simulink model "KDO"  (R2017b)
settings: Solver=FixedStepAuto  StartTime=0.0  StopTime=100  FixedStep=0.001  RelTol=1e-3
undefined symbols (not defined in the file or in its folder): B, k1, k2, k3, k4, k5, k6, MI
libraries: powerlib_extras x15, commchan3 x15, simulink x3, checkpacklib x1
(part 1 of 3)
settings Model: Creator=Jose_Canche  LastModifiedBy=nuradeen
settings DataIOCC: LimitDataPoints=on  SaveFormat=Array
settings OptimizationCC: ExpressionDepthLimit=2147483647  InitFltsAndDblsToZero=on  LifeSpan=inf
settings DebuggingCC: SaveWithParameterizedLinksMsg=none  UnderspecifiedInitializationDetection=Classic  MergeDetectMultiDrivingBlocksExec=none  SolverPrmCheckMsg=warning  FcnCallInpInsideContextMsg=warning  StateNameClashWarn=warning  SFUnexpectedBacktrackingDiag=warning  SFNoUnconditionalDefaultTransitionDiag=warning  SFExecutionAtInitializationDiag=none
settings HardwareCC: ProdBitPerPointer=32  ProdBitPerSizeT=32  ProdBitPerPtrDiffT=32  ProdLargestAtomicFloat=None  ProdIntDivRoundTo=Undefined  ProdEndianess=Unspecified  ProdWordSize=32  ProdHWDeviceType=32-bit Generic
settings ModelReferenceCC: PropagateSignalLabelsOutOfModel=off
settings SFSimCC: SimParseCustomCode=off
settings CodeAppCC: StateflowObjectComments=on
settings GRTTargetCC: TargetFcnLib=ansi_tfl_tmw.mat  TargetLangStandard=C89/C90 (ANSI)  GeneratePreprocessorConditionals=Disable all  CombineOutputUpdateFcns=off  GRTInterface=on
settings ConfigComp: CovMetricSettings=dw  CovHtmlReporting=on  CovSaveCumulativeToWorkspaceVar=on  CovSaveSingleToWorkspaceVar=on  CovExternalEMLEnable=off  CovSFcnEnable=off
settings SimscapeCC: SimscapeNormalizeSystem=off
settings ConfigurationSet: Description=SimMechanics 2G

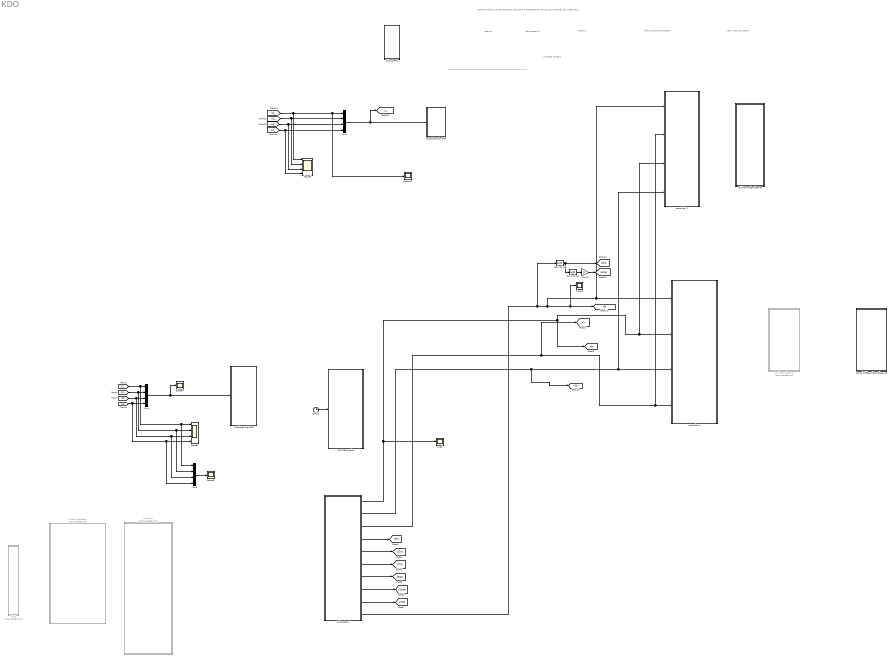
== system KDO ==
  note: -----------------------------------------------------------------------------------------------------------------------
  note: Parameters IC
  note: clear all
  note: Graphs
  note: NDO and sliding mode observers Applied to a QUADROTOR
      | (comparison between two observers)
  note: compare controls
  note: KDO: Disturbance Graphs
  note: KDO: Tracking Graphs
  " sliding mode observer " : Subsystem
  " Quadrotor Plant #2" : Subsystem
  " Quadrotor plant #1 " : Subsystem
  " Kernel Differentiator Observer" : Subsystem
  " Nonlinear Observer " : Subsystem  Commented=on
  Clock3 : Clock
  Derivative2 : Derivative
  Derivative3 : Derivative
  Gain3 : Gain  Gain=0
  MATLAB Function : MATLAB Function  TreatAsAtomicUnit=on
  Mux1 : Mux
  Mux4 : Mux
  Mux5 : Mux
  Scope{,2,4,13} (4 alike) : Scope
  Scope3 : Scope  NumInputPorts=4
  Scope5 : Scope  NumInputPorts=4
  Subsystem1 : Subsystem
  Subsystem2 : Subsystem
  Traj3 : Subsystem  Commented=on
  Trajectory : Subsystem  Commented=on
  Valeurs désirées1 : Subsystem  Commented=on
  controller  1 : Subsystem
  controller 2 : Subsystem
  "x_ref " : Scope
  tag scope: U_=global, x11r=global, x11rp=global, x11rpp=global, x5r=global, x5rp=global, x5rpp=global, x7r=global, x7rp=global, x7rpp=global, x9r=global, x9rp=global, x9rpp=global
  wires:
  [U4_] -> Scope5/4, Mux1/4
  [U3_] -> Scope5/3, Mux1/3
  [U1_] -> Scope5/1, Mux1/1, Scope13/1
  [U2_] -> Scope5/2, Mux1/2
  Mux1/1 -> [U_], " Quadrotor plant #1 "/1(In1)
  Subsystem2/1(x) -> "x_ref "/1, controller  1/3(In3), controller 2/2(In2), [x9r]
  Subsystem2/2(y) -> [x11r], controller  1/4(In4), controller 2/3(In3)
  Subsystem2/3(z) -> [x7r], controller  1/2(In2), controller 2/4(In4)
  Mux4/1 -> Scope4/1, " Quadrotor Plant #2"/1(In1)
  [U1] -> Mux5/1, Scope3/1, Mux4/1
  [U2] -> Mux5/2, Scope3/2, Mux4/2
  [U3] -> Mux5/3, Scope3/3, Mux4/3
  [U4] -> Mux5/4, Scope3/4, Mux4/4
  Mux5/1 -> Scope2/1
  Subsystem2/10(yaw) -> Derivative3/1, controller  1/1(In1), controller 2/1(In1), [x5r], Scope/1
  Derivative2/1 -> Gain3/1
  Gain3/1 -> [x5rpp]
  Derivative3/1 -> [x5rp], Derivative2/1
  Clock3/1 -> MATLAB Function/1(t)
  Subsystem2/4(dx) -> [x9rp]
  Subsystem2/5("dy ") -> [x11rp]
  Subsystem2/6(dz) -> [x7rp]
  Subsystem2/7(ddx) -> [x9rpp]
  Subsystem2/8(ddy) -> [x11rpp]
  Subsystem2/9(ddz) -> [x7rpp]

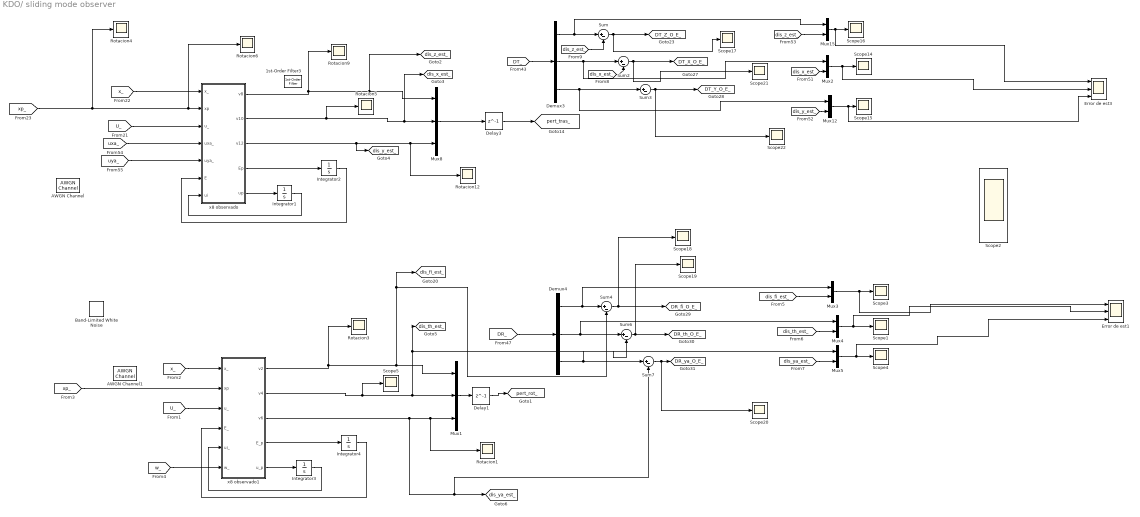
== system KDO/ sliding mode observer  ==
  1st-Order Filter3 : powerlib_extras/Control  Blocks/1st-Order  Filter  FilterType=Lowpass  Tc=5  Initialize=off  Vac_Init=[0.8 -25 60]  Vdc_Init=-0.4  PlotResponse=off  param1=[1 500 1]
  AWGN Channel : commchan3/AWGN Channel  InputProcessing=Columns as channels (frame based)  seed=67  noiseMode="Signal to noise ratio  (SNR)"  EbNodB=10  EsNodB=10  SNRdB=20  bitsPerSym=1  Ps=10  Tsym=1  variance=1
      settings: SourceProductName=Communications Toolbox
  AWGN Channel1 : commchan3/AWGN Channel  InputProcessing=Columns as channels (frame based)  seed=67  noiseMode="Signal to noise ratio  (SNR)"  EbNodB=10  EsNodB=10  SNRdB=20  bitsPerSym=1  Ps=10  Tsym=1  variance=1
      settings: SourceProductName=Communications Toolbox
  Band-Limited White Noise : simulink/Sources/Band-Limited White Noise  Cov=[1]  Ts=1  seed=[23341]
  Delay1 : Delay  DelayLength=1  InitialCondition=0
  Delay3 : Delay  DelayLength=1  InitialCondition=0
  Demux3 : Demux  Outputs=3
  Demux4 : Demux  Outputs=3
  Error de est1 : Scope  NumInputPorts=3
  Error de est3 : Scope  NumInputPorts=3
  Integrator{1..4} (4 alike) : Integrator  InitialCondition=[0 0 0];
  Mux1 : Mux  Inputs=3
  Mux{2..5,12,15} (6 alike) : Mux  Inputs=2
  Mux8 : Mux  Inputs=3
  Rotacion{1,3..6,9,12} (7 alike) : Scope
  Scope{1,3..5,14..22} (13 alike) : Scope
  Scope2 : Scope  NumInputPorts=3
  Sum{,2..4,6..7} (6 alike) : Sum  Inputs=|+-
  x8 observado : MATLAB Function  TreatAsAtomicUnit=on
  x8 observado1 : MATLAB Function  TreatAsAtomicUnit=on
  tag scope: DR_fi_O_E_=global, DR_th_O_E_=global, DR_ya_O_E_=global, DT_X_O_E_=global, DT_Y_O_E_=global, DT_Z_O_E_=global, dis_fi_est_=global, dis_th_est_=global, dis_x_est_=global, dis_y_est_=global, dis_ya_est_=global, dis_z_est_=global, pert_rot_=global, pert_tras_=global
  wires:
  Integrator2/1 -> x8 observado/6(E)
  Integrator1/1 -> x8 observado/7(ui)
  Mux8/1 -> Delay3/1
  x8 observado/5(up) -> Integrator1/1
  x8 observado/4(Ep) -> Integrator2/1
  [x_] -> x8 observado/1(x_)
  [U_] -> x8 observado/3(u_)
  [uya_] -> x8 observado/5(uya_)
  [uxa_] -> x8 observado/4(uxa_)
  Integrator4/1 -> x8 observado1/4(E_)
  Integrator3/1 -> x8 observado1/5(ui_)
  Delay1/1 -> [pert_rot_]
  x8 observado1/5(u_p) -> Integrator3/1
  x8 observado1/4(E_p) -> Integrator4/1
  [x_] -> x8 observado1/1(x_)
  [U_] -> x8 observado1/3(u_)
  Mux1/1 -> Delay1/1
  [w_] -> x8 observado1/6(w_)
  [dis_y_est_] -> Mux12/2
  Sum3/1 -> [DT_Y_O_E_], Scope22/1
  Mux15/1 -> Error de est3/1, Scope16/1
  Mux12/1 -> Error de est3/3, Scope15/1
  Demux3/3 -> Mux12/1, Sum3/1
  [dis_x_est_] -> Mux2/2
  Demux3/1 -> Mux15/1, Sum/1
  Sum2/1 -> [DT_X_O_E_], Scope21/1
  Mux2/1 -> Error de est3/2, Scope14/1
  [DT_] -> Demux3/1
  [dis_z_est_] -> Mux15/2
  Demux3/2 -> Mux2/1, Sum2/1
  Sum/1 -> [DT_Z_O_E_], Scope17/1
  Sum6/1 -> Scope19/1, [DR_th_O_E_]
  Sum4/1 -> Scope18/1, [DR_fi_O_E_]
  Sum7/1 -> Scope20/1, [DR_ya_O_E_]
  Demux4/3 -> Mux5/1, Sum7/1
  Demux4/2 -> Mux4/1, Sum6/1
  [DR_] -> Demux4/1
  Mux3/1 -> Error de est1/1, Scope3/1
  Demux4/1 -> Mux3/1, Sum4/1
  [dis_fi_est_] -> Mux3/2
  Mux4/1 -> Error de est1/2, Scope1/1
  [dis_th_est_] -> Mux4/2
  Mux5/1 -> Error de est1/3, Scope4/1
  [dis_ya_est_] -> Mux5/2
  [dis_x_est_] -> Sum2/2
  Delay3/1 -> [pert_tras_]
  x8 observado/1(v8) -> Rotacion9/1, [dis_z_est_], Mux8/1
  x8 observado/2(v10) -> Rotacion5/1, [dis_x_est_], Mux8/2
  x8 observado/3(v12) -> [dis_y_est_], Rotacion12/1, Mux8/3
  [dis_z_est_] -> Sum/2
  x8 observado1/1(v2) -> Rotacion3/1, Sum4/2, [dis_fi_est_], Mux1/1
  x8 observado1/2(v4) -> Scope5/1, [dis_th_est_], Sum6/2, Mux1/2
  x8 observado1/3(v6) -> Sum7/2, [dis_ya_est_], Rotacion1/1, Mux1/3
  [xp_] -> Rotacion4/1, Rotacion6/1, x8 observado/2(xp)
  [xp_] -> x8 observado1/2(xp)

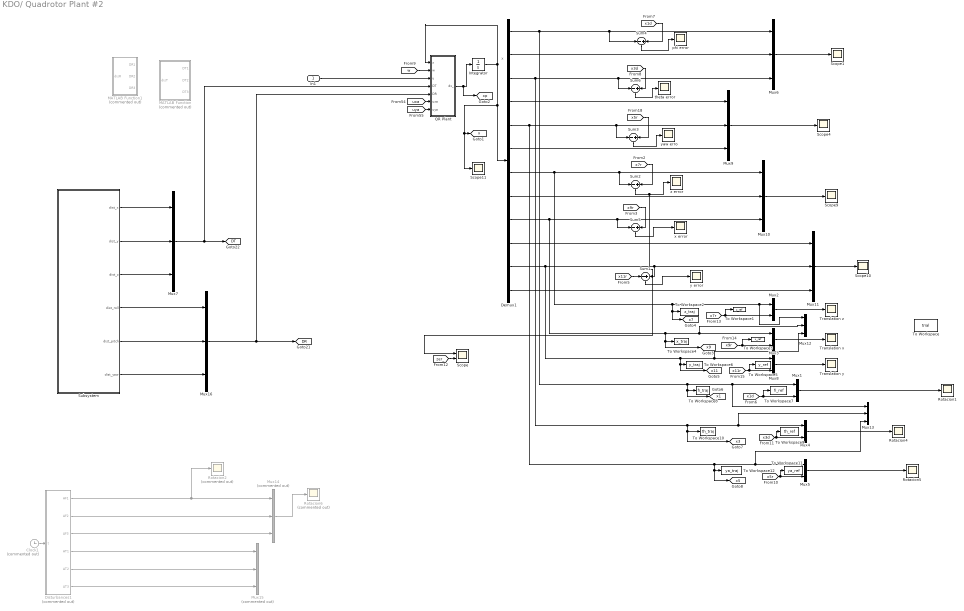
== system KDO/ Quadrotor Plant #2 ==
  note: x
  In1 : Inport
  Clock1 : Clock  Commented=on
  Demux1 : Demux  Outputs=12
  Disturbances1 : MATLAB Function  Commented=on  TreatAsAtomicUnit=on
  Integrator : Integrator  InitialCondition=[0 0 0 0 0 0 0 0 0 0 0 0];
  MATLAB Function : MATLAB Function  Commented=on  TreatAsAtomicUnit=on
  MATLAB Function1 : MATLAB Function  Commented=on  TreatAsAtomicUnit=on
  Mux{1..5,8} (6 alike) : Mux  Inputs=2
  Mux{6..7,9..13,16} (8 alike) : Mux  Inputs=3
  Mux14 : Mux  Commented=on  Inputs=3
  Mux15 : Mux  Commented=on  Inputs=3
  "QR Plant " : MATLAB Function  TreatAsAtomicUnit=on
  Rotacion1 : Scope
  Rotacion2 : Scope  Commented=on
  Rotacion4 : Scope
  Rotacion5 : Scope
  Rotacion6 : Scope  Commented=on
  Scope : Scope  NumInputPorts=2
  Scope{1,4,9..11} (5 alike) : Scope
  Subsystem : Subsystem
  Sum{1..6} (6 alike) : Sum  Inputs=-+
  To Workspace : ToWorkspace  VariableName=trial  SaveFormat=Timeseries  SampleTime=-1
  To Workspace1 : ToWorkspace  VariableName=z_ref  SaveFormat=Timeseries  SampleTime=-1
  To Workspace10 : ToWorkspace  VariableName=th_traj  SaveFormat=Timeseries  SampleTime=-1
  To Workspace11 : ToWorkspace  VariableName=ya_ref  SaveFormat=Timeseries  SampleTime=-1
  To Workspace12 : ToWorkspace  VariableName=ya_traj  SaveFormat=Timeseries  SampleTime=-1
  To Workspace2 : ToWorkspace  VariableName=z_traj  SaveFormat=Timeseries  SampleTime=-1
  To Workspace3 : ToWorkspace  VariableName=x_ref  SaveFormat=Timeseries  SampleTime=-1
  To Workspace4 : ToWorkspace  VariableName=x_traj  SaveFormat=Timeseries  SampleTime=-1
  To Workspace5 : ToWorkspace  VariableName=y_ref  SaveFormat=Timeseries  SampleTime=-1
  To Workspace6 : ToWorkspace  VariableName=y_traj  SaveFormat=Timeseries  SampleTime=-1
  To Workspace7 : ToWorkspace  VariableName=fi_ref  SaveFormat=Timeseries  SampleTime=-1
  To Workspace8 : ToWorkspace  VariableName=fi_traj  SaveFormat=Timeseries  SampleTime=-1
  To Workspace9 : ToWorkspace  VariableName=th_ref  SaveFormat=Timeseries  SampleTime=-1
  "Translation x " : Scope
  "Translation y " : Scope
  "Translation z " : Scope
  phi error : Scope
  theta error : Scope
  x error : Scope
  "y error " : Scope
  yaw erro : Scope
  z error : Scope
  tag scope: DR=global, DT=global, x11=global, x1=global, x3=global, x5=global, x7=global, x9=global, x=global, xp=global
  wires:
  Mux6/1 -> Scope1/1
  In1/1 -> "QR Plant "/3(u)
  Mux11/1 -> Scope10/1
  Demux1/2 -> Mux6/2
  Demux1/12 -> Mux11/3
  Demux1/1 -> To Workspace8/1, [x1], Mux13/1, Mux1/1, Sum4/1, Mux6/1
  [w] -> "QR Plant "/2(w)
  Demux1/3 -> [x3], To Workspace10/1, Mux13/2, Mux4/1, Sum6/1, Mux6/3
  Mux10/1 -> Scope9/1
  Demux1/4 -> Mux9/1
  Demux1/10 -> Mux11/1
  Mux9/1 -> Scope4/1
  Demux1/8 -> Mux10/2
  Demux1/6 -> Mux9/3
  Demux1/5 -> To Workspace12/1, [x5], Mux13/3, Mux5/1, Sum3/1, Mux9/2
  Sum4/1 -> phi error/1
  Sum6/1 -> theta error/1
  Sum3/1 -> yaw erro/1
  Demux1/7 -> Mux12/1, Mux2/1, [x7], To Workspace2/1, Sum2/1, Mux10/1
  Sum2/1 -> z error/1, Scope/1
  Demux1/9 -> [x9], To Workspace4/1, Mux12/2, Mux3/1, Sum5/1, Mux10/3
  Sum5/1 -> x error/1
  Demux1/11 -> [x11], To Workspace6/1, Mux12/3, Mux8/1, Sum1/2, Mux11/2
  [x11r] -> Sum1/1
  Sum1/1 -> "y error "/1
  [x1d] -> Sum4/2
  [x1d] -> To Workspace7/1, Mux1/2
  [x3d] -> To Workspace9/1, Mux4/2
  [x5r] -> To Workspace11/1, Mux5/2
  Mux5/1 -> Rotacion5/1
  Mux4/1 -> Rotacion4/1
  Mux1/1 -> Rotacion1/1
  [uxa] -> "QR Plant "/6(uxa)
  [uya] -> "QR Plant "/7(uya)
  Integrator/1 -> "QR Plant "/1(x), Scope11/1, [x], Demux1/1
  [zer_] -> Scope/2
  [x7r] -> To Workspace1/1, Mux2/2
  [x9r] -> To Workspace3/1, Mux3/2
  [x11r] -> To Workspace5/1, Mux8/2
  Mux3/1 -> "Translation x "/1
  Mux8/1 -> "Translation y "/1
  Mux2/1 -> "Translation z "/1
  "QR Plant "/1(dx_) -> [xp], Integrator/1
  [x5r] -> Sum3/2
  [x7r] -> Sum2/2
  [x9r] -> Sum5/2
  [x3d] -> Sum6/2
  Disturbances1/1(AF1) -> Rotacion2/1, Mux14/1
  Clock1/1 -> Disturbances1/1(t)
  Disturbances1/6(AT3) -> Mux15/3
  Disturbances1/3(AF3) -> Mux14/3
  Disturbances1/4(AT1) -> Mux15/1
  Disturbances1/5(AT2) -> Mux15/2
  Disturbances1/2(AF2) -> Mux14/2
  Mux14/1 -> Rotacion6/1
  Mux16/1 -> [DR], "QR Plant "/5(DR)
  Subsystem/6(dist_yaw) -> Mux16/3
  Subsystem/4(dist_roll) -> Mux16/1
  Subsystem/5(dist_pitch) -> Mux16/2
  Subsystem/2(dist_y) -> Mux7/2
  Subsystem/3(dist_z) -> Mux7/3
  Subsystem/1(dist_x) -> Mux7/1
  Mux7/1 -> [DT], "QR Plant "/4(DT)

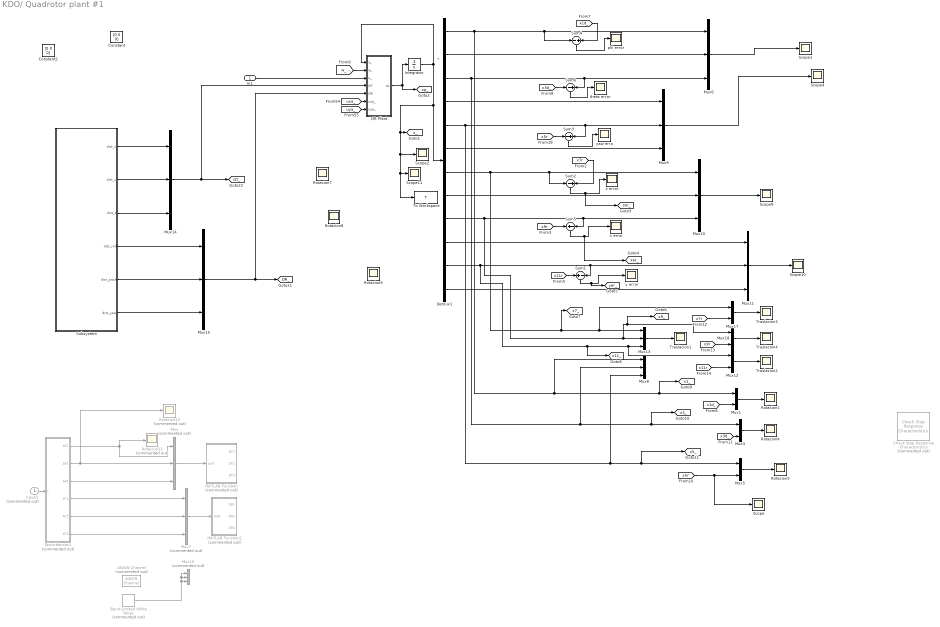
== system KDO/ Quadrotor plant #1  ==
  note: x
  In1 : Inport
  AWGN Channel : commchan3/AWGN Channel  Commented=on  InputProcessing=Columns as channels (frame based)  seed=67  noiseMode="Signal to noise ratio  (SNR)"  EbNodB=10  EsNodB=10  SNRdB=20  bitsPerSym=1  Ps=1  Tsym=1  variance=1
      settings: SourceProductName=Communications Toolbox
  Band-Limited White Noise : simulink/Sources/Band-Limited White Noise  Commented=on  Cov=[1]  Ts=1  seed=[23341]
  Check Step Response Characteristics : checkpacklib/Check Step Response  Characteristics  Commented=on  InstantiateOnLoad=on  enabled=on  stopWhenAssertionFail=off  export=off  ViewDlgPos=[]  OpenViewOnLoad=off  LaunchViewOnOpen=off  TimeUnits=seconds  EnableStepResponseBound=on  InitialValue=0  FinalValue=1  StepTime=0  RiseTime=3  PercentRise=80  SettlingTime=7  PercentSettling=1  PercentOvershoot=5  PercentUndershoot=1
  Clock1 : Clock  Commented=on
  Constant : Constant  Value=[0 0 0]
  Constant2 : Constant  Value=[0 0 0]
  Demux1 : Demux  Outputs=12
  Disturbances1 : MATLAB Function  Commented=on  TreatAsAtomicUnit=on
  Integrator : Integrator  InitialCondition=[0 0 0 0 0 0 0 0 0 0 0 0];
  MATLAB Function : MATLAB Function  Commented=on  TreatAsAtomicUnit=on
  MATLAB Function1 : MATLAB Function  Commented=on  TreatAsAtomicUnit=on
  Mux : Mux  Commented=on  Inputs=3
  Mux{1,4..5,12,17..18} (6 alike) : Mux  Inputs=2
  Mux{6,8..11,13..15} (8 alike) : Mux  Inputs=3
  Mux16 : Mux  Commented=on  Inputs=3
  Mux7 : Mux  Commented=on  Inputs=3
  "QR Plant " : MATLAB Function  TreatAsAtomicUnit=on
  Rotacion{1,4..5,7..9} (6 alike) : Scope
  Rotacion10 : Scope  Commented=on
  Rotacion11 : Scope  Commented=on
  Scope{,1..2,4,9..11} (7 alike) : Scope
  Subsystem : Subsystem
  Sum1 : Sum  Inputs=+-
  Sum{2..4,6} (4 alike) : Sum  Inputs=-+
  Sum5 : Sum  Inputs=+-
  To Workspace : ToWorkspace  VariableName=T  SaveFormat=Timeseries  SampleTime=-1
  Traslacion{1..4} (4 alike) : Scope
  phi error : Scope
  theta error : Scope
  x error : Scope
  "y error " : Scope
  yaw erro : Scope
  z error : Scope
  tag scope: DR_=global, DT_=global, x11_=global, x1_=global, x3_=global, x5_=global, x7_=global, x9_=global, x_=global, xer_=global, xp_=global, yer_=global, zer_=global
  wires:
  Clock1/1 -> Disturbances1/1(t)
  Integrator/1 -> Scope2/1, To Workspace/1, Scope11/1, [x_], Demux1/1, "QR Plant "/1(x_)
  Mux6/1 -> Scope1/1
  In1/1 -> "QR Plant "/3(u_)
  Mux11/1 -> Scope10/1
  Demux1/1 -> Mux8/1, [x1_], Mux1/1, Sum4/1, Mux6/1
  Mux13/1 -> Traslacion1/1
  [w_] -> "QR Plant "/2(w_)
  "QR Plant "/1(dx) -> [xp_], Integrator/1
  Demux1/3 -> Mux8/2, [x3_], Mux4/1, Sum6/2, Mux6/3
  Mux10/1 -> Scope9/1
  Mux9/1 -> Scope4/1
  Demux1/5 -> Mux8/3, [x5_], Mux5/1, Sum3/2, Mux9/2
  Sum4/1 -> phi error/1
  [x3d_] -> Sum6/1
  Sum6/1 -> theta error/1
  Sum3/1 -> yaw erro/1
  [x5r] -> Sum3/1
  Demux1/7 -> [x7_], Mux17/1, Mux13/1, Sum2/1, Mux10/1
  Sum2/1 -> [zer_], z error/1
  Demux1/9 -> [x9_], Mux18/1, Mux13/2, Sum5/2, Mux10/3
  Sum5/1 -> [xer_], x error/1
  [x9r] -> Sum5/1
  Demux1/11 -> Sum1/2, Mux11/2, [x11_], Mux12/1, Mux13/3
  [x11r] -> Sum1/1
  Sum1/1 -> [yer_], "y error "/1
  [x1d_] -> Sum4/2
  [x1d_] -> Mux1/2
  [x3d_] -> Mux4/2
  [x5r] -> Scope/1, Mux5/2
  Mux5/1 -> Rotacion5/1
  Mux4/1 -> Rotacion4/1
  Mux1/1 -> Rotacion1/1
  [uxa_] -> "QR Plant "/6(uxa_)
  [uya_] -> "QR Plant "/7(uya_)
  [x7r] -> Sum2/2
  Disturbances1/2(AF2) -> Rotacion10/1, Mux/2
  Disturbances1/5(AT2) -> Mux7/2
  Disturbances1/6(AT3) -> Mux7/3
  Mux12/1 -> Traslacion2/1
  Mux7/1 -> MATLAB Function1/1(disR)
  Disturbances1/4(AT1) -> Mux7/1
  Disturbances1/3(AF3) -> Mux/3
  Disturbances1/1(AF1) -> Rotacion11/1, Mux/1
  Band-Limited White Noise/1 -> Mux16/2, Mux16/1, Mux16/3
  [x7r] -> Mux17/2
  [x9r] -> Mux18/2
  [x11r] -> Mux12/2
  Mux18/1 -> Traslacion4/1
  Mux17/1 -> Traslacion3/1
  Demux1/2 -> Mux6/2
  Demux1/4 -> Mux9/1
  Demux1/6 -> Mux9/3
  Demux1/8 -> Mux10/2
  Demux1/10 -> Mux11/1
  Demux1/12 -> Mux11/3
  Mux/1 -> MATLAB Function/1(disT)
  Subsystem/1(dist_x) -> Mux14/1
  Subsystem/2(dist_y) -> Mux14/2
  Subsystem/3(dist_z) -> Mux14/3
  Mux14/1 -> "QR Plant "/4(DT), [DT_]
  Subsystem/4(dist_roll) -> Mux15/1
  Subsystem/5(dist_pitch) -> Mux15/2
  Subsystem/6(dist_yaw) -> Mux15/3
  Mux15/1 -> "QR Plant "/5(DR), [DR_]

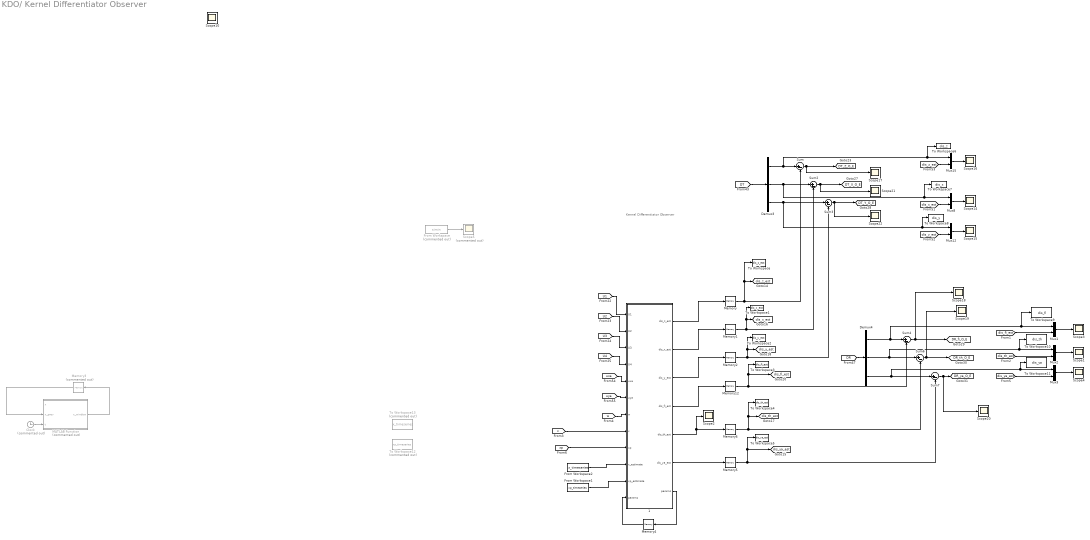
== system KDO/ Kernel Differentiator Observer ==
  note: Kernel Differentiator
      | Observer
  " 1" : MATLAB Function  TreatAsAtomicUnit=on
  Clock : Clock  Commented=on
  Demux3 : Demux  Outputs=3
  Demux4 : Demux  Outputs=3
  From Workspace : FromWorkspace  Commented=on  VariableName=simin  SampleTime=0
  From Workspace1 : FromWorkspace  VariableName=xp_timeseries
  From Workspace2 : FromWorkspace  VariableName=x_timeseries  SampleTime=0
  MATLAB Function : MATLAB Function  Commented=on  TreatAsAtomicUnit=on
  Memory{,1..2,5..6,12} (6 alike) : Memory
  Memory3 : Memory  Commented=on  InitialCondition=zeros(51,7)
  Memory4 : Memory  InitialCondition=ones(4,6)
  Mux{1..3,8,12,15} (6 alike) : Mux  Inputs=2
  Scope{1..4,10,14..22} (14 alike) : Scope
  Scope5 : Scope  Commented=on
  Sum{,2..4,6..7} (6 alike) : Sum  Inputs=|+-
  To Workspace : ToWorkspace  VariableName=dis_z_est  SaveFormat=Timeseries  SampleTime=-1
  To Workspace1 : ToWorkspace  VariableName=dis_x_est  SaveFormat=Timeseries  SampleTime=-1
  To Workspace10 : ToWorkspace  VariableName=dis_th  SaveFormat=Timeseries  SampleTime=-1
  To Workspace11 : ToWorkspace  VariableName=dis_ya  SaveFormat=Timeseries  SampleTime=-1
  To Workspace12 : ToWorkspace  Commented=on  VariableName=xp_timeseries  SaveFormat=Timeseries  SampleTime=-1
  To Workspace13 : ToWorkspace  Commented=on  VariableName=x_timeseries  SaveFormat=Timeseries  SampleTime=-1
  To Workspace2 : ToWorkspace  VariableName=dis_y_est  SaveFormat=Timeseries  SampleTime=-1
  To Workspace3 : ToWorkspace  VariableName=dis_fi_est  SaveFormat=Timeseries  SampleTime=-1
  To Workspace4 : ToWorkspace  VariableName=dis_th_est  SaveFormat=Timeseries  SampleTime=-1
  To Workspace5 : ToWorkspace  VariableName=dis_ya_est  SaveFormat=Timeseries  SampleTime=-1
  To Workspace6 : ToWorkspace  VariableName=dis_z  SaveFormat=Timeseries  SampleTime=-1
  To Workspace7 : ToWorkspace  VariableName=dis_x  SaveFormat=Timeseries  SampleTime=-1
  To Workspace8 : ToWorkspace  VariableName=dis_y  SaveFormat=Timeseries  SampleTime=-1
  To Workspace9 : ToWorkspace  VariableName=dis_fi  SaveFormat=Timeseries  SampleTime=-1
  tag scope: DR_fi_O_E=global, DR_th_O_E=global, DR_ya_O_E=global, DT_X_O_E=global, DT_Y_O_E=global, DT_Z_O_E=global, dis_fi_est=global, dis_th_est=global, dis_x_est=global, dis_y_est=global, dis_ya_est=global, dis_z_est=global
  wires:
  [dis_fi_est] -> Mux1/2
  " 1"/6(dis_ya_est) -> Memory5/1
  Demux4/1 -> To Workspace9/1, Mux1/1, Sum4/1
  " 1"/3(dis_y_est) -> Memory2/1
  Demux4/2 -> To Workspace10/1, Mux2/1, Sum6/1
  [U2] -> " 1"/2(U2)
  Memory/1 -> To Workspace/1, [dis_z_est], Sum/2
  [DT] -> Demux3/1
  " 1"/1(dis_z_est) -> Memory/1
  " 1"/2(dis_x_est) -> Memory1/1
  [dis_z_est] -> Mux15/2
  Sum6/1 -> Scope19/1, [DR_th_O_E]
  Memory6/1 -> To Workspace4/1, [dis_th_est], Sum6/2
  " 1"/5(dis_th_est) -> Memory6/1, Scope2/1
  Mux1/1 -> Scope3/1
  Memory2/1 -> To Workspace2/1, [dis_y_est], Sum3/2
  Mux3/1 -> Scope4/1
  Memory1/1 -> Sum2/2, To Workspace1/1, [dis_x_est]
  Memory5/1 -> Sum7/2, To Workspace5/1, [dis_ya_est]
  Demux3/2 -> To Workspace7/1, Mux8/1, Sum2/1
  Mux8/1 -> Scope14/1
  Memory12/1 -> Sum4/2, To Workspace3/1, [dis_fi_est]
  Sum/1 -> [DT_Z_O_E], Scope17/1
  [dis_th_est] -> Mux2/2
  Sum4/1 -> Scope18/1, [DR_fi_O_E]
  Sum7/1 -> Scope20/1, [DR_ya_O_E]
  [U4] -> " 1"/4(U4)
  Demux4/3 -> To Workspace11/1, Mux3/1, Sum7/1
  [dis_ya_est] -> Mux3/2
  Sum2/1 -> [DT_X_O_E], Scope21/1
  Demux3/3 -> To Workspace8/1, Mux12/1, Sum3/1
  Demux3/1 -> To Workspace6/1, Mux15/1, Sum/1
  [DR] -> Demux4/1
  Mux12/1 -> Scope15/1
  [U1] -> " 1"/1(U1)
  [dis_x_est] -> Mux8/2
  Sum3/1 -> [DT_Y_O_E], Scope22/1
  Mux2/1 -> Scope1/1
  " 1"/4(dis_fi_est) -> Memory12/1
  [U3] -> " 1"/3(U3)
  [w] -> " 1"/7(w)
  Mux15/1 -> Scope16/1
  [dis_y_est] -> Mux12/2
  MATLAB Function/1(x_window) -> Memory3/1
  Memory3/1 -> MATLAB Function/2(x_prev)
  [uya] -> " 1"/6(uya)
  [uxa] -> " 1"/5(uxa)
  " 1"/7(params) -> Memory4/1
  Memory4/1 -> " 1"/12("params ")
  Clock/1 -> MATLAB Function/3(t)
  [xp] -> " 1"/9(xp)
  [x] -> " 1"/8(x)
  From Workspace/1 -> Scope5/1
  From Workspace2/1 -> " 1"/10(x_estimate)
  From Workspace1/1 -> " 1"/11(xp_estimate)

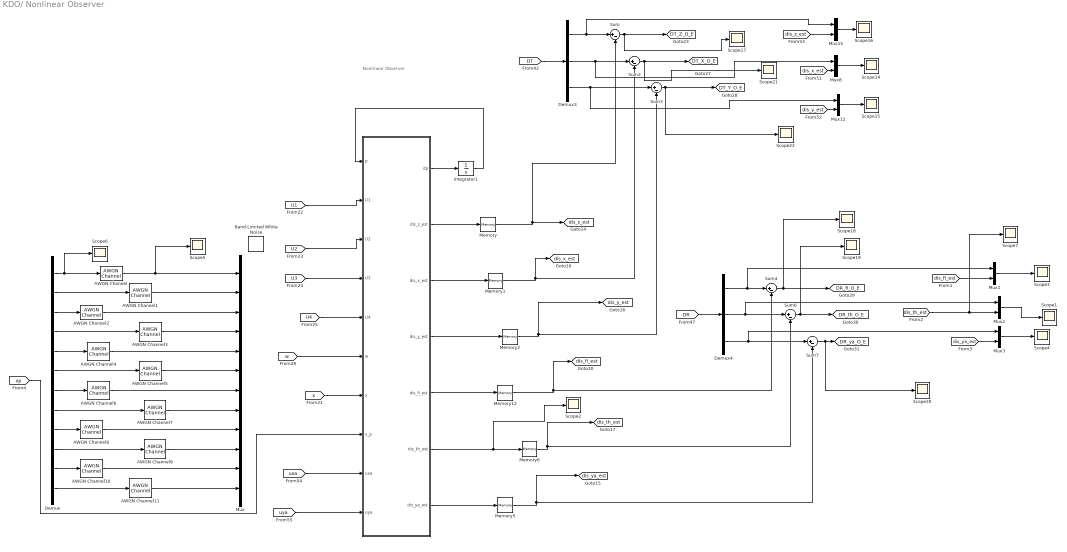
== system KDO/ Nonlinear Observer  ==
  note: Nonlinear Observer
  " " : MATLAB Function  TreatAsAtomicUnit=on
  AWGN Channel{,1..7,9..11} (11 alike) : commchan3/AWGN Channel  InputProcessing=Columns as channels (frame based)  seed=67  noiseMode="Signal to noise ratio  (SNR)"  EbNodB=10  EsNodB=10  SNRdB=20  bitsPerSym=1  Ps=1  Tsym=1  variance=1
      settings: SourceProductName=Communications Toolbox
  AWGN Channel8 : commchan3/AWGN Channel  InputProcessing=Columns as channels (frame based)  seed=67  noiseMode="Signal to noise ratio  (SNR)"  EbNodB=40  EsNodB=10  SNRdB=20  bitsPerSym=1  Ps=1  Tsym=1  variance=1
      settings: SourceProductName=Communications Toolbox
  Band-Limited White Noise : simulink/Sources/Band-Limited White Noise  Cov=[0.1]  Ts=0.1  seed=[23341]
  Demux : Demux  Outputs=12
  Demux3 : Demux  Outputs=3
  Demux4 : Demux  Outputs=3
  Integrator1 : Integrator  InitialCondition=[0 0 0 0 0 0];
  Memory{,1..2,5..6,12} (6 alike) : Memory
  Mux : Mux  Inputs=12
  Mux{1..3,8,12,15} (6 alike) : Mux  Inputs=2
  Scope{1..7,14..22} (16 alike) : Scope
  Sum{,2..4,6..7} (6 alike) : Sum  Inputs=|+-
  tag scope: DR_fi_O_E=global, DR_th_O_E=global, DR_ya_O_E=global, DT_X_O_E=global, DT_Y_O_E=global, DT_Z_O_E=global, dis_fi_est=global, dis_th_est=global, dis_x_est=global, dis_y_est=global, dis_ya_est=global, dis_z_est=global
  wires:
  [dis_y_est] -> Mux12/2
  Integrator1/1 -> " "/1(p)
  Sum6/1 -> Scope19/1, [DR_th_O_E]
  Sum3/1 -> [DT_Y_O_E], Scope22/1
  Mux15/1 -> Scope16/1
  Mux12/1 -> Scope15/1
  [w] -> " "/6(w)
  Sum4/1 -> Scope18/1, [DR_fi_O_E]
  Demux3/3 -> Mux12/1, Sum3/1
  Sum7/1 -> Scope20/1, [DR_ya_O_E]
  [dis_x_est] -> Mux8/2
  Demux3/1 -> Mux15/1, Sum/1
  Sum2/1 -> [DT_X_O_E], Scope21/1
  Demux4/3 -> Mux3/1, Sum7/1
  Mux8/1 -> Scope14/1
  Demux4/2 -> Mux2/1, Sum6/1
  [DT] -> Demux3/1
  [dis_z_est] -> Mux15/2
  Demux3/2 -> Mux8/1, Sum2/1
  [DR] -> Demux4/1
  [U1] -> " "/2(U1)
  [U2] -> " "/3(U2)
  [U3] -> " "/4(U3)
  [U4] -> " "/5(U4)
  Sum/1 -> [DT_Z_O_E], Scope17/1
  [uxa] -> " "/9(uxa)
  [uya] -> " "/10(uya)
  " "/1(dp) -> Integrator1/1
  Memory5/1 -> Sum7/2, [dis_ya_est]
  Memory6/1 -> [dis_th_est], Sum6/2
  Mux1/1 -> Scope3/1
  Demux4/1 -> Mux1/1, Sum4/1
  [dis_fi_est] -> Mux1/2
  Mux2/1 -> Scope1/1
  Mux3/1 -> Scope4/1
  [dis_ya_est] -> Mux3/2
  [dis_th_est] -> Scope7/1, Mux2/2
  [x] -> " "/7(x)
  Demux/1 -> Scope6/1, AWGN Channel/1
  Demux/2 -> AWGN Channel1/1
  Demux/3 -> AWGN Channel2/1
  Demux/4 -> AWGN Channel3/1
  Demux/5 -> AWGN Channel4/1
  Demux/6 -> AWGN Channel5/1
  Demux/7 -> AWGN Channel6/1
  Demux/8 -> AWGN Channel7/1
  Demux/9 -> AWGN Channel8/1
  Demux/10 -> AWGN Channel9/1
  Demux/11 -> AWGN Channel10/1
  Demux/12 -> AWGN Channel11/1
  AWGN Channel/1 -> Scope5/1, Mux/1
  AWGN Channel1/1 -> Mux/2
  AWGN Channel2/1 -> Mux/3
  AWGN Channel3/1 -> Mux/4
  AWGN Channel4/1 -> Mux/5
  AWGN Channel5/1 -> Mux/6
  AWGN Channel6/1 -> Mux/7
  AWGN Channel7/1 -> Mux/8
  AWGN Channel8/1 -> Mux/9
  AWGN Channel9/1 -> Mux/10
  AWGN Channel10/1 -> Mux/11
  AWGN Channel11/1 -> Mux/12
  Memory/1 -> Sum/2, [dis_z_est]
  Memory1/1 -> Sum2/2, [dis_x_est]
  Memory2/1 -> Sum3/2, [dis_y_est]
  Memory12/1 -> Sum4/2, [dis_fi_est]
  " "/2(dis_z_est) -> Memory/1
  " "/3(dis_x_est) -> Memory1/1
  " "/4(dis_y_est) -> Memory2/1
  " "/5(dis_fi_est) -> Memory12/1
  " "/6(dis_th_est) -> Scope2/1, Memory6/1
  " "/7(dis_ya_est) -> Memory5/1
  [xp] -> " "/8(x_p)

== system KDO/Subsystem1 ==
  Mux{,2..3,6..8} (6 alike) : Mux  Inputs=3
  Scope : Scope
  Scope1 : Scope  NumInputPorts=3
  Scope2 : Scope
  Scope3 : Scope
  Scope6 : Scope  NumInputPorts=3
  wires:
  Mux6/1 -> Scope6/1
  [x5] -> Mux6/2
  [x5r] -> Mux6/1
  [x1d] -> Mux7/1
  [x3d] -> Mux8/1
  [x5_] -> Mux6/3
  [x3_] -> Mux8/3
  [x1_] -> Mux7/3
  [x3] -> Mux8/2
  [x1] -> Mux7/2
  [x9r] -> Mux/1
  [x9] -> Mux/2
  [x9_] -> Mux/3
  [x7_] -> Mux2/3
  [x7r] -> Mux2/1
  [x7] -> Mux2/2
  [x11_] -> Mux3/3
  [x11r] -> Mux3/1
  [x11] -> Mux3/2
  Mux/1 -> Scope/1, Scope1/1
  Mux3/1 -> Scope3/1, Scope1/2
  Mux2/1 -> Scope2/1, Scope1/3
  Mux7/1 -> Scope6/2
  Mux8/1 -> Scope6/3

== system KDO/Subsystem2 ==
  Clock1 : Clock
  Scope1 : Scope  NumInputPorts=3
  xyz _desired1 : MATLAB Function  TreatAsAtomicUnit=on
  x : Outport
  y : Outport  Port=2
  z : Outport  Port=3
  dx : Outport  Port=4
  "dy " : Outport  Port=5
  dz : Outport  Port=6
  ddx : Outport  Port=7
  ddy : Outport  Port=8
  ddz : Outport  Port=9
  yaw : Outport  Port=10
  wires:
  xyz _desired1/4(dx) -> dx/1
  Clock1/1 -> xyz _desired1/1(t)
  xyz _desired1/1(x) -> x/1, Scope1/1
  xyz _desired1/3(z) -> z/1, Scope1/3
  xyz _desired1/2(y) -> Scope1/2, y/1
  xyz _desired1/5(dy) -> "dy "/1
  xyz _desired1/6(dz) -> dz/1
  xyz _desired1/7(ddx) -> ddx/1
  xyz _desired1/8(ddy) -> ddy/1
  xyz _desired1/9(ddz) -> ddz/1
  xyz _desired1/10(yaw) -> yaw/1

== system KDO/Traj3 ==
  Clock : Clock
  Clock1 : Clock
  Constant : Constant  Value=0
  Gain : Gain  Gain=0.1
  Mux : Mux  Inputs=3
  Scope3 : Scope  NumInputPorts=3
  Subsystem : Subsystem
  To Workspace : ToWorkspace  VariableName=xyzd1  SampleTime=-1
  Trajectory : MATLAB Function  TreatAsAtomicUnit=on
  xyz _desired : MATLAB Function  TreatAsAtomicUnit=on
  x : Outport
  ddx : Outport  Port=2
  y : Outport  Port=3
  ddy : Outport  Port=4
  z : Outport  Port=5
  ddz : Outport  Port=6
  yaw : Outport  Port=7
  wires:
  Constant/1 -> yaw/1
  Clock/1 -> xyz _desired/1(t)
  Mux/1 -> To Workspace/1
  Trajectory/1(qi) -> Mux/3, Scope3/3, z/1
  Clock1/1 -> Trajectory/1(t)
  Trajectory/3(qidd) -> ddz/1
  Trajectory/2(qid) -> ?
  xyz _desired/2(ddx) -> ddx/1
  xyz _desired/4(ddy) -> ddy/1
  xyz _desired/1(x) -> x/1, Mux/1, Scope3/1
  xyz _desired/3(y) -> Scope3/2, Mux/2, y/1

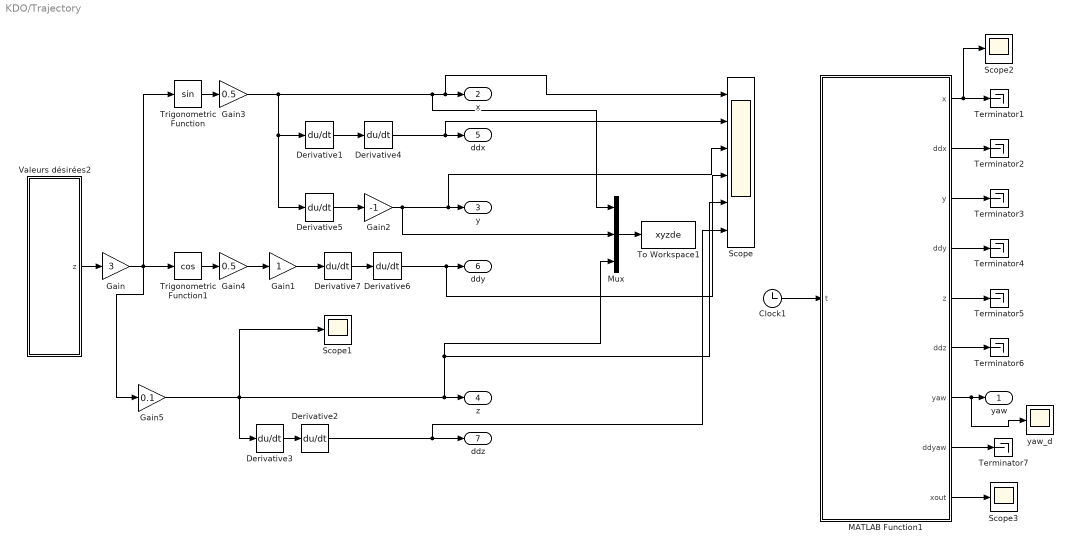
== system KDO/Trajectory ==
  Clock1 : Clock
  Derivative{1..7} (7 alike) : Derivative
  Gain : Gain  Gain=3
  Gain1 : Gain
  Gain2 : Gain  Gain=-1
  Gain3 : Gain  Gain=0.5
  Gain4 : Gain  Gain=0.5
  Gain5 : Gain  Gain=0.1
  MATLAB Function1 : MATLAB Function  TreatAsAtomicUnit=on
  Mux : Mux  Inputs=3
  Scope : Scope  NumInputPorts=6
  Scope1 : Scope
  Scope2 : Scope
  Scope3 : Scope
  Terminator{1..7} (7 alike) : Terminator
  To Workspace1 : ToWorkspace  VariableName=xyzde  SampleTime=-1
  Trigonometric Function : Trigonometry
  Trigonometric Function1 : Trigonometry  Operator=cos
  Valeurs désirées2 : Subsystem
  yaw_d : Scope
  yaw : Outport
  x : Outport  Port=2
  y : Outport  Port=3
  z : Outport  Port=4
  ddx : Outport  Port=5
  ddy : Outport  Port=6
  ddz : Outport  Port=7
  wires:
  Clock1/1 -> MATLAB Function1/1(t)
  MATLAB Function1/1(x) -> Scope2/1, Terminator1/1
  MATLAB Function1/2(ddx) -> Terminator2/1
  MATLAB Function1/3(y) -> Terminator3/1
  MATLAB Function1/4(ddy) -> Terminator4/1
  MATLAB Function1/5(z) -> Terminator5/1
  MATLAB Function1/6(ddz) -> Terminator6/1
  MATLAB Function1/7(yaw) -> yaw_d/1, yaw/1
  MATLAB Function1/8(ddyaw) -> Terminator7/1
  MATLAB Function1/9(xout) -> Scope3/1
  Derivative1/1 -> Derivative4/1
  Valeurs désirées2/1(z) -> Gain/1
  Derivative3/1 -> Derivative2/1
  Mux/1 -> To Workspace1/1
  Derivative2/1 -> Scope/6, ddz/1
  Derivative4/1 -> Scope/2, ddx/1
  Trigonometric Function/1 -> Gain3/1
  Gain/1 -> Gain5/1, Trigonometric Function1/1, Trigonometric Function/1
  Derivative6/1 -> Scope/4, ddy/1
  Derivative5/1 -> Gain2/1
  Derivative7/1 -> Derivative6/1
  Gain1/1 -> Derivative7/1
  Trigonometric Function1/1 -> Gain4/1
  Gain2/1 -> Mux/2, Scope/3, y/1
  Gain3/1 -> Mux/1, Scope/1, x/1, Derivative5/1, Derivative1/1
  Gain4/1 -> Gain1/1
  Gain5/1 -> Scope1/1, Derivative3/1, Scope/5, Mux/3, z/1

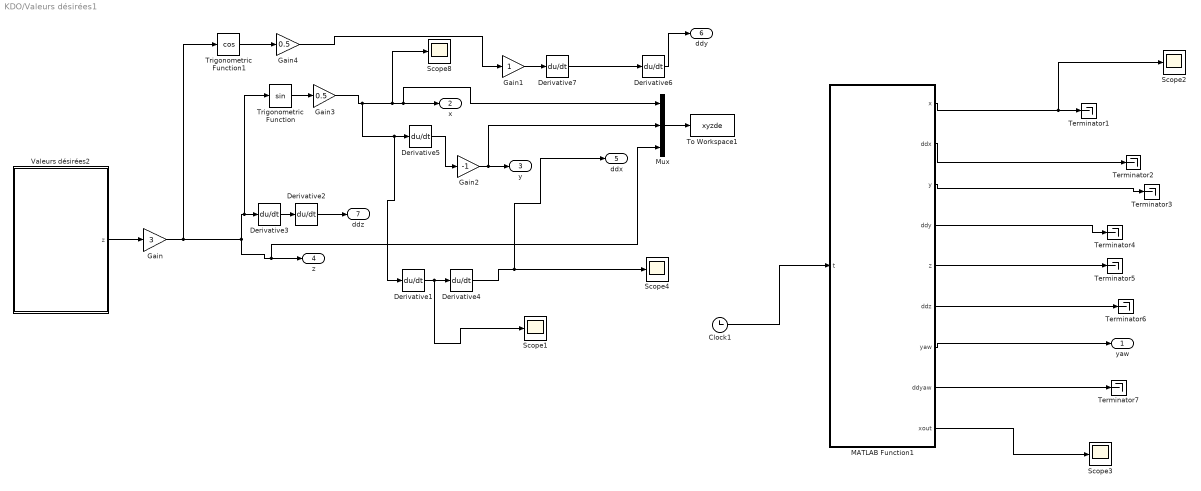
== system KDO/Valeurs désirées1 ==
  Clock1 : Clock
  Derivative{1..7} (7 alike) : Derivative
  Gain : Gain  Gain=3
  Gain1 : Gain
  Gain2 : Gain  Gain=-1
  Gain3 : Gain  Gain=0.5
  Gain4 : Gain  Gain=0.5
  MATLAB Function1 : MATLAB Function  TreatAsAtomicUnit=on
  Mux : Mux  Inputs=3
  Scope{1..4,8} (5 alike) : Scope
  Terminator{1..7} (7 alike) : Terminator
  To Workspace1 : ToWorkspace  VariableName=xyzde  SampleTime=-1
  Trigonometric Function : Trigonometry
  Trigonometric Function1 : Trigonometry  Operator=cos
  Valeurs désirées2 : Subsystem
  yaw : Outport
  x : Outport  Port=2
  y : Outport  Port=3
  z : Outport  Port=4
  ddx : Outport  Port=5
  ddy : Outport  Port=6
  ddz : Outport  Port=7
  wires:
  Clock1/1 -> MATLAB Function1/1(t)
  MATLAB Function1/1(x) -> Scope2/1, Terminator1/1
  MATLAB Function1/2(ddx) -> Terminator2/1
  MATLAB Function1/3(y) -> Terminator3/1
  MATLAB Function1/4(ddy) -> Terminator4/1
  MATLAB Function1/5(z) -> Terminator5/1
  MATLAB Function1/6(ddz) -> Terminator6/1
  MATLAB Function1/7(yaw) -> yaw/1
  MATLAB Function1/8(ddyaw) -> Terminator7/1
  MATLAB Function1/9(xout) -> Scope3/1
  Derivative1/1 -> Scope1/1, Derivative4/1
  Valeurs désirées2/1(z) -> Gain/1
  Derivative3/1 -> Derivative2/1
  Mux/1 -> To Workspace1/1
  Derivative2/1 -> ddz/1
  Derivative4/1 -> ddx/1, Scope4/1
  Trigonometric Function/1 -> Gain3/1
  Gain/1 -> Trigonometric Function1/1, Mux/3, z/1, Trigonometric Function/1, Derivative3/1
  Derivative6/1 -> ddy/1
  Derivative5/1 -> Gain2/1
  Derivative7/1 -> Derivative6/1
  Gain1/1 -> Derivative7/1
  Trigonometric Function1/1 -> Gain4/1
  Gain2/1 -> Mux/2, y/1
  Gain3/1 -> Derivative5/1, Derivative1/1, Scope8/1, Mux/1, x/1
  Gain4/1 -> Gain1/1

== system KDO/controller  1 ==
  In1 : Inport
  In2 : Inport  Port=2
  In3 : Inport  Port=3
  In4 : Inport  Port=4
  " angular velocity calculation" : Subsystem
  " Rotational control" : Subsystem
  Position controller : Subsystem
  wires:
  In1/1 -> Position controller/1(In1)
  In2/1 -> Position controller/2(In2)
  In3/1 -> Position controller/3(In3)
  In4/1 -> Position controller/4(In4)

== system KDO/controller 2 ==
  In1 : Inport
  In2 : Inport  Port=2
  In3 : Inport  Port=3
  In4 : Inport  Port=4
  " angular velocity calculation" : Subsystem
  Position controller : Subsystem
  "Rotational controller " : Subsystem
  wires:
  In1/1 -> Position controller/1(In1)
  In2/1 -> Position controller/2(In2)
  In3/1 -> Position controller/3(In3)
  In4/1 -> Position controller/4(In4)

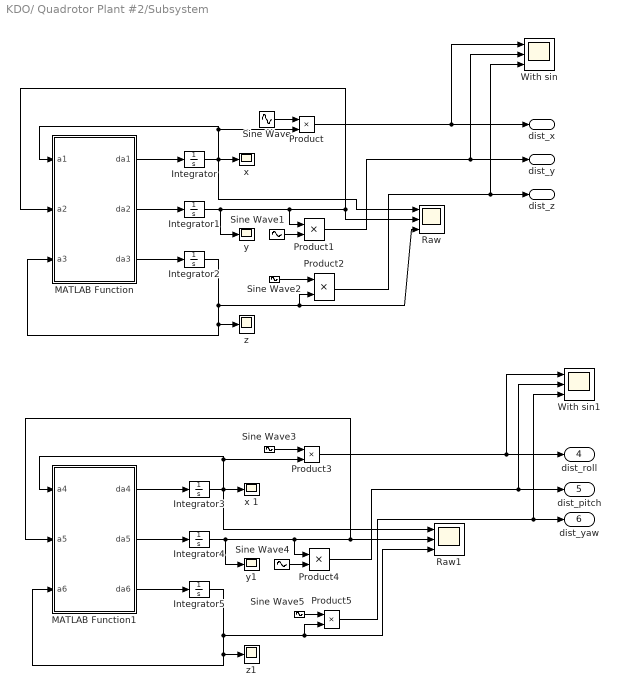
== system KDO/ Quadrotor Plant #2/Subsystem ==
  Integrator : Integrator  InitialCondition=0.1
  Integrator1 : Integrator  InitialCondition=3
  Integrator2 : Integrator  InitialCondition=0.5
  Integrator3 : Integrator  InitialCondition=5
  Integrator4 : Integrator  InitialCondition=-5
  Integrator5 : Integrator  InitialCondition=10
  MATLAB Function : MATLAB Function  TreatAsAtomicUnit=on
  MATLAB Function1 : MATLAB Function  TreatAsAtomicUnit=on
  Product{,1..5} (6 alike) : Product
  Raw : Scope  NumInputPorts=3
  Raw1 : Scope  NumInputPorts=3
  Sine Wave : Sin  Amplitude=0.01  Phase=-20  SampleTime=0
  Sine Wave1 : Sin  Amplitude=0.01  Phase=-40  SampleTime=0
  Sine Wave2 : Sin  Amplitude=0.01  Phase=-60  SampleTime=0
  Sine Wave3 : Sin  Amplitude=0.01  Phase=-15  SampleTime=0
  Sine Wave4 : Sin  Amplitude=0.01  Phase=-35  SampleTime=0
  Sine Wave5 : Sin  Amplitude=0.01  Phase=-55  SampleTime=0
  With sin : Scope  NumInputPorts=3
  With sin1 : Scope  NumInputPorts=3
  "x " : Scope
  x 1 : Scope
  y : Scope
  y1 : Scope
  z : Scope
  z1 : Scope
  dist_x : Outport
  dist_y : Outport  Port=2
  dist_z : Outport  Port=3
  dist_roll : Outport  Port=4
  dist_pitch : Outport  Port=5
  dist_yaw : Outport  Port=6
  wires:
  MATLAB Function1/2(da5) -> Integrator4/1
  Sine Wave3/1 -> Product3/1
  Sine Wave4/1 -> Product4/2
  Product5/1 -> With sin1/3, dist_yaw/1
  Sine Wave5/1 -> Product5/1
  Integrator4/1 -> Product4/1, MATLAB Function1/2(a5), Raw1/2, y1/1
  Integrator/1 -> Raw/1, MATLAB Function/1(a1), Product/2, "x "/1
  Sine Wave/1 -> Product/1
  Integrator3/1 -> Raw1/1, MATLAB Function1/1(a4), Product3/2, x 1/1
  MATLAB Function/3(da3) -> Integrator2/1
  MATLAB Function1/1(da4) -> Integrator3/1
  Product3/1 -> With sin1/1, dist_roll/1
  MATLAB Function1/3(da6) -> Integrator5/1
  Product4/1 -> With sin1/2, dist_pitch/1
  Integrator1/1 -> Product1/1, MATLAB Function/2(a2), Raw/2, y/1
  MATLAB Function/2(da2) -> Integrator1/1
  MATLAB Function/1(da1) -> Integrator/1
  Integrator2/1 -> Product2/2, Raw/3, MATLAB Function/3(a3), z/1
  Sine Wave2/1 -> Product2/1
  Sine Wave1/1 -> Product1/2
  Product2/1 -> With sin/3, dist_z/1
  Product/1 -> With sin/1, dist_x/1
  Product1/1 -> With sin/2, dist_y/1
  Integrator5/1 -> Product5/2, Raw1/3, MATLAB Function1/3(a6), z1/1

== system KDO/ Quadrotor plant #1 /Subsystem ==
  Integrator : Integrator  InitialCondition=0.1
  Integrator1 : Integrator  InitialCondition=3
  Integrator2 : Integrator  InitialCondition=0.5
  Integrator3 : Integrator  InitialCondition=5
  Integrator4 : Integrator  InitialCondition=-5
  Integrator5 : Integrator  InitialCondition=10
  MATLAB Function : MATLAB Function  TreatAsAtomicUnit=on
  MATLAB Function1 : MATLAB Function  TreatAsAtomicUnit=on
  Product{,1..5} (6 alike) : Product
  Raw : Scope  NumInputPorts=3
  Raw1 : Scope  NumInputPorts=3
  Sine Wave : Sin  Amplitude=0.01  Phase=-20  SampleTime=0
  Sine Wave1 : Sin  Amplitude=0.01  Phase=-40  SampleTime=0
  Sine Wave2 : Sin  Amplitude=0.01  Phase=-60  SampleTime=0
  Sine Wave3 : Sin  Amplitude=0.01  Phase=-15  SampleTime=0
  Sine Wave4 : Sin  Amplitude=0.01  Phase=-35  SampleTime=0
  Sine Wave5 : Sin  Amplitude=0.01  Phase=-55  SampleTime=0
  With sin : Scope  NumInputPorts=3
  With sin1 : Scope  NumInputPorts=3
  "x " : Scope
  x 1 : Scope
  y : Scope
  y1 : Scope
  z : Scope
  z1 : Scope
  dist_x : Outport
  dist_y : Outport  Port=2
  dist_z : Outport  Port=3
  dist_roll : Outport  Port=4
  dist_pitch : Outport  Port=5
  dist_yaw : Outport  Port=6
  wires:
  MATLAB Function1/2(da5) -> Integrator4/1
  Sine Wave3/1 -> Product3/1
  Sine Wave4/1 -> Product4/2
  Product5/1 -> With sin1/3, dist_yaw/1
  Sine Wave5/1 -> Product5/1
  Integrator4/1 -> Product4/1, MATLAB Function1/2(a5), Raw1/2, y1/1
  Integrator/1 -> Raw/1, MATLAB Function/1(a1), Product/2, "x "/1
  Sine Wave/1 -> Product/1
  Integrator3/1 -> Raw1/1, MATLAB Function1/1(a4), Product3/2, x 1/1
  MATLAB Function/3(da3) -> Integrator2/1
  MATLAB Function1/1(da4) -> Integrator3/1
  Product3/1 -> With sin1/1, dist_roll/1
  MATLAB Function1/3(da6) -> Integrator5/1
  Product4/1 -> With sin1/2, dist_pitch/1
  Integrator1/1 -> Product1/1, MATLAB Function/2(a2), Raw/2, y/1
  MATLAB Function/2(da2) -> Integrator1/1
  MATLAB Function/1(da1) -> Integrator/1
  Integrator2/1 -> Product2/2, Raw/3, MATLAB Function/3(a3), z/1
  Sine Wave2/1 -> Product2/1
  Sine Wave1/1 -> Product1/2
  Product2/1 -> With sin/3, dist_z/1
  Product/1 -> With sin/1, dist_x/1
  Product1/1 -> With sin/2, dist_y/1
  Integrator5/1 -> Product5/2, Raw1/3, MATLAB Function1/3(a6), z1/1

== system KDO/Traj3/Subsystem ==
  Clock : Clock
  xyz _desired : MATLAB Function  TreatAsAtomicUnit=on
  z : Outport
  wires:
  xyz _desired/3(z) -> z/1
  Clock/1 -> xyz _desired/1(t)

== system KDO/Trajectory/Valeurs désirées2 ==
  Clock : Clock
  MATLAB Function : MATLAB Function  TreatAsAtomicUnit=on
  Scope6 : Scope
  Scope8 : Scope
  Terminator1 : Terminator
  Terminator11 : Terminator
  z : Outport
  wires:
  Clock/1 -> MATLAB Function/1(t)
  MATLAB Function/1(x) -> Terminator11/1
  MATLAB Function/2(y) -> Terminator1/1
  MATLAB Function/3(z) -> z/1, Scope6/1
  MATLAB Function/4(xout) -> Scope8/1

== system KDO/Valeurs désirées1/Valeurs désirées2 ==
  Clock : Clock
  MATLAB Function : MATLAB Function  TreatAsAtomicUnit=on
  Scope6 : Scope
  Scope8 : Scope
  Terminator1 : Terminator
  Terminator11 : Terminator
  z : Outport
  wires:
  Clock/1 -> MATLAB Function/1(t)
  MATLAB Function/1(x) -> Terminator11/1
  MATLAB Function/2(y) -> Terminator1/1
  MATLAB Function/3(z) -> z/1, Scope6/1
  MATLAB Function/4(xout) -> Scope8/1

== system KDO/controller  1/ angular velocity calculation ==
  1st-Order Filter{8..11} (4 alike) : powerlib_extras/Control  Blocks/1st-Order  Filter  FilterType=Lowpass  Tc=5  Initialize=off  Vac_Init=[0.8 -25 60]  Vdc_Init=-0.4  PlotResponse=off  param1=[1 500 1]
  Constant1 : Constant  Value=MI
  Constant6 : Constant  Value=B
  Demux1 : Demux
  Demux2 : Demux
  Demux9 : Demux
  Divide2 : Product  Inputs=**  Multiplication=Matrix(*)
  Divide6 : Product  Inputs=**  Multiplication=Matrix(*)
  Math Function : Math  Operator=sqrt  SaturateOnIntegerOverflow=on
  Math Function1 : Math  Operator=sqrt  SaturateOnIntegerOverflow=on
  Memory5 : Memory
  Mux4 : Mux
  Scope23 : Scope  NumInputPorts=4
  Scope4 : Scope  NumInputPorts=4
  Scope6 : Scope
  Sum1 : Sum  Inputs=+-+-
  tag scope: w_=global
  wires:
  Math Function/1 -> Scope6/1, Demux2/1
  [U4_] -> Mux4/4
  Demux2/4 -> Sum1/4
  [U1_] -> Mux4/1
  [U3_] -> Mux4/3
  [U2_] -> Mux4/2
  Sum1/1 -> [w_]
  Constant1/1 -> Divide2/1
  Demux2/2 -> Sum1/2
  Demux2/3 -> Sum1/3
  Demux2/1 -> Sum1/1
  Mux4/1 -> Divide2/2
  Memory5/1 -> Math Function/1
  Constant6/1 -> Divide6/1
  Demux9/1 -> Scope23/1
  Demux9/2 -> Scope23/2
  Demux9/3 -> Scope23/3
  Demux9/4 -> Scope23/4
  Divide6/1 -> Math Function1/1
  Demux1/1 -> 1st-Order Filter8/1
  Demux1/2 -> 1st-Order Filter9/1
  Demux1/3 -> 1st-Order Filter10/1
  Demux1/4 -> 1st-Order Filter11/1
  Divide2/1 -> Memory5/1, Demux1/1, Divide6/2
  1st-Order Filter8/1 -> Scope4/1
  1st-Order Filter9/1 -> Scope4/2
  1st-Order Filter10/1 -> Scope4/3
  1st-Order Filter11/1 -> Scope4/4
  Math Function1/1 -> Demux9/1

== system KDO/controller  1/ Rotational control ==
  Constant : Constant  Value=[0 0 0]
  Constant{15..18} (4 alike) : Constant  Value=0
  Derivative : Derivative
  Derivative1 : Derivative
  Rotational Control : MATLAB Function  TreatAsAtomicUnit=on
  Rotational Control1 : MATLAB Function  Commented=on  TreatAsAtomicUnit=on
  Scope1 : Scope
  Scope2 : Scope
  Scope3 : Scope
  tag scope: U2_=global, U3_=global, U4_=global
  wires:
  [x5rpp] -> Rotational Control/4(x5rpp)
  Rotational Control/3(U4_) -> Scope3/1, [U4_]
  [x5r] -> Rotational Control/2(x5r)
  [x5rp] -> Rotational Control/3(x5rp)
  [w_] -> Rotational Control/5(w)
  Rotational Control/1(U2_) -> Scope1/1, [U2_]
  Rotational Control/2(U3_) -> Scope2/1, [U3_]
  Constant18/1 -> Rotational Control/8(x1dpp)
  [x_] -> Rotational Control/1(x)
  [x1d_] -> Derivative/1, Rotational Control/6(x1d)
  [x3d_] -> Derivative1/1, Rotational Control/9(x3d)
  Constant15/1 -> Rotational Control/11(x3dpp)
  Derivative/1 -> Rotational Control/7(x1dp)
  Derivative1/1 -> Rotational Control/10(x3dp)
  [pert_rot_] -> Rotational Control/12(pert_rot_)

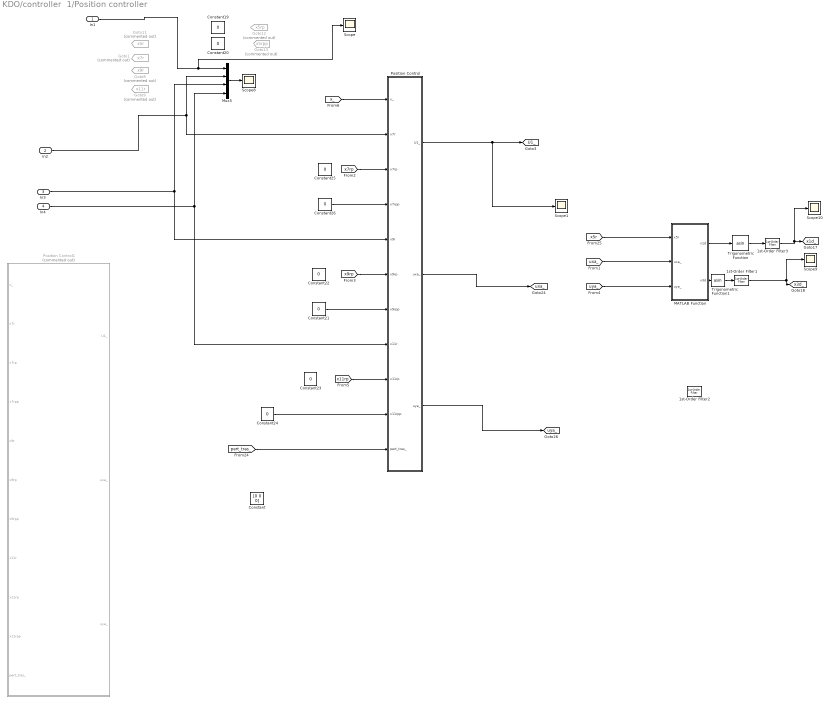
== system KDO/controller  1/Position controller ==
  In1 : Inport
  In2 : Inport  Port=2
  In3 : Inport  Port=3
  In4 : Inport  Port=4
  1st-Order Filter1 : powerlib_extras/Control  Blocks/1st-Order  Filter  FilterType=Lowpass  Tc=5  Initialize=off  Vac_Init=[0.8 -25 60]  Vdc_Init=-0.4  PlotResponse=off  param1=[1 500 1]
  1st-Order Filter2 : powerlib_extras/Control  Blocks/1st-Order  Filter  FilterType=Lowpass  Tc=5  Initialize=off  Vac_Init=[0.8 -25 60]  Vdc_Init=-0.4  PlotResponse=off  param1=[1 500 1]
  1st-Order Filter3 : powerlib_extras/Control  Blocks/1st-Order  Filter  FilterType=Lowpass  Tc=5  Initialize=off  Vac_Init=[0.8 -25 60]  Vdc_Init=-0.4  PlotResponse=off  param1=[1 500 1]
  Constant : Constant  Value=[0 0 0]
  Constant{19..26} (8 alike) : Constant  Value=0
  Goto1 : Goto  Commented=on  GotoTag=x7r  TagVisibility=global
  Goto11 : Goto  Commented=on  GotoTag=x5r  TagVisibility=global
  Goto12 : Goto  Commented=on  GotoTag=x5rp  TagVisibility=global
  Goto13 : Goto  Commented=on  GotoTag=x5rpp  TagVisibility=global
  Goto8 : Goto  Commented=on  GotoTag=x9r  TagVisibility=global
  Goto9 : Goto  Commented=on  GotoTag=x11r  TagVisibility=global
  MATLAB Function : MATLAB Function  TreatAsAtomicUnit=on
  Mux5 : Mux
  Position Control : MATLAB Function  TreatAsAtomicUnit=on
  Position Control1 : MATLAB Function  Commented=on  TreatAsAtomicUnit=on
  Scope{,1,8..10} (5 alike) : Scope
  Trigonometric Function : Trigonometry  Operator=asin
  Trigonometric Function1 : Trigonometry  Operator=asin
  tag scope: U1_=global, uxa_=global, uya_=global, x1d_=global, x3d_=global
  wires:
  In3/1 -> Position Control/5(x9r), Mux5/3
  In4/1 -> Position Control/8(x11r), Mux5/4
  [x5r] -> MATLAB Function/1(x5r)
  MATLAB Function/1(x1d) -> Trigonometric Function/1
  Trigonometric Function1/1 -> 1st-Order Filter1/1
  Trigonometric Function/1 -> 1st-Order Filter3/1
  [uxa_] -> MATLAB Function/2(uxa_)
  [uya_] -> MATLAB Function/3(uya_)
  Mux5/1 -> Scope8/1
  Constant24/1 -> Position Control/10(x11rpp)
  Constant26/1 -> Position Control/4(x7rpp)
  In1/1 -> Scope/1, Mux5/1
  Position Control/3(uya_) -> [uya_]
  Position Control/1(U1_) -> Scope1/1, [U1_]
  Position Control/2(uxa_) -> [uxa_]
  In2/1 -> Position Control/2(x7r), Mux5/2
  [x_] -> Position Control/1(x_)
  Constant21/1 -> Position Control/7(x9rpp)
  MATLAB Function/2(x3d) -> Trigonometric Function1/1
  1st-Order Filter3/1 -> Scope10/1, [x1d_]
  [x7rp] -> Position Control/3(x7rp)
  [x9rp] -> Position Control/6(x9rp)
  [x11rp] -> Position Control/9(x11rp)
  1st-Order Filter1/1 -> Scope9/1, [x3d_]
  [pert_tras_] -> Position Control/11(pert_tras_)

== system KDO/controller 2/ angular velocity calculation ==
  1st-Order Filter{8..11} (4 alike) : powerlib_extras/Control  Blocks/1st-Order  Filter  FilterType=Lowpass  Tc=5  Initialize=off  Vac_Init=[0.8 -25 60]  Vdc_Init=-0.4  PlotResponse=off  param1=[1 500 1]
  Constant1 : Constant  Value=MI
  Constant6 : Constant  Value=B
  Delay : Delay  DelayLength=1  InitialCondition=0
  Demux1 : Demux
  Demux2 : Demux
  Demux9 : Demux
  Divide2 : Product  Inputs=**  Multiplication=Matrix(*)
  Divide6 : Product  Inputs=**  Multiplication=Matrix(*)
  Math Function : Math  Operator=sqrt  SaturateOnIntegerOverflow=on
  Math Function1 : Math  Operator=sqrt  SaturateOnIntegerOverflow=on
  Mux4 : Mux
  Scope1 : Scope
  Scope2 : Scope
  Scope23 : Scope  NumInputPorts=4
  Scope4 : Scope  NumInputPorts=4
  Scope6 : Scope
  Sum1 : Sum  Inputs=++--
  tag scope: w=global
  wires:
  Math Function/1 -> Scope6/1, Demux2/1
  [U4] -> Mux4/4
  Demux2/4 -> Sum1/4
  [U1] -> Mux4/1
  [U3] -> Mux4/3
  [U2] -> Mux4/2
  Sum1/1 -> Delay/1
  Constant1/1 -> Divide2/1
  Demux2/2 -> Sum1/2
  Demux2/3 -> Sum1/3
  Demux2/1 -> Sum1/1
  Mux4/1 -> Divide2/2
  Divide2/1 -> Math Function/1, Demux1/1, Divide6/2
  Constant6/1 -> Divide6/1
  Demux9/1 -> Scope1/1, Scope23/1
  Demux9/2 -> Scope23/2
  Demux9/3 -> Scope23/3
  Demux9/4 -> Scope23/4
  Divide6/1 -> Math Function1/1
  Demux1/1 -> 1st-Order Filter8/1
  Demux1/2 -> 1st-Order Filter9/1
  Demux1/3 -> 1st-Order Filter10/1
  Demux1/4 -> 1st-Order Filter11/1
  1st-Order Filter8/1 -> Scope4/1
  1st-Order Filter9/1 -> Scope4/2
  1st-Order Filter10/1 -> Scope4/3
  1st-Order Filter11/1 -> Scope4/4
  Math Function1/1 -> Demux9/1
  Delay/1 -> Scope2/1, [w]

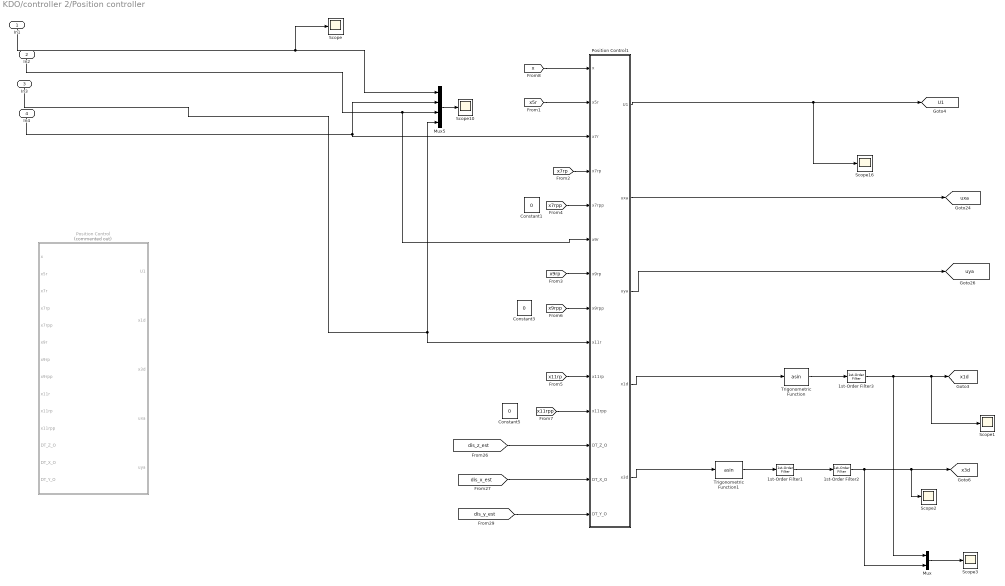
== system KDO/controller 2/Position controller ==
  In1 : Inport
  In2 : Inport  Port=2
  In3 : Inport  Port=3
  In4 : Inport  Port=4
  1st-Order Filter1 : powerlib_extras/Control  Blocks/1st-Order  Filter  FilterType=Lowpass  Tc=5  Initialize=off  Vac_Init=[0.8 -25 60]  Vdc_Init=-0.4  PlotResponse=off  param1=[1 500 1]
  1st-Order Filter2 : powerlib_extras/Control  Blocks/1st-Order  Filter  FilterType=Lowpass  Tc=5  Initialize=off  Vac_Init=[0.8 -25 60]  Vdc_Init=-0.4  PlotResponse=off  param1=[1 500 1]
  1st-Order Filter3 : powerlib_extras/Control  Blocks/1st-Order  Filter  FilterType=Lowpass  Tc=5  Initialize=off  Vac_Init=[0.8 -25 60]  Vdc_Init=-0.4  PlotResponse=off  param1=[1 500 1]
  Constant1 : Constant  Value=0
  Constant3 : Constant  Value=0
  Constant5 : Constant  Value=0
  Mux : Mux  Inputs=2
  Mux5 : Mux
  Position Control : MATLAB Function  Commented=on  TreatAsAtomicUnit=on
  Position Control1 : MATLAB Function  TreatAsAtomicUnit=on
  Scope{,1..3,10,16} (6 alike) : Scope
  Trigonometric Function : Trigonometry  Operator=asin
  Trigonometric Function1 : Trigonometry  Operator=asin
  tag scope: U1=global, uxa=global, uya=global, x1d=global, x3d=global
  wires:
  In2/1 -> Position Control1/6(x9r), Mux5/3
  In3/1 -> Position Control1/9(x11r), Mux5/4
  In4/1 -> Position Control1/3(x7r), Mux5/2
  In1/1 -> Scope/1, Mux5/1
  Position Control1/5(x3d) -> Trigonometric Function1/1
  Position Control1/4(x1d) -> Trigonometric Function/1
  Position Control1/1(U1) -> Scope16/1, [U1]
  [x] -> Position Control1/1(x)
  Mux5/1 -> Scope10/1
  Position Control1/2(uxa) -> [uxa]
  Position Control1/3(uya) -> [uya]
  Trigonometric Function/1 -> 1st-Order Filter3/1
  Trigonometric Function1/1 -> 1st-Order Filter1/1
  [x5r] -> Position Control1/2(x5r)
  1st-Order Filter3/1 -> Mux/1, Scope1/1, [x1d]
  1st-Order Filter1/1 -> 1st-Order Filter2/1
  1st-Order Filter2/1 -> Mux/2, Scope2/1, [x3d]
  [x7rp] -> Position Control1/4(x7rp)
  [x9rp] -> Position Control1/7(x9rp)
  [x11rp] -> Position Control1/10(x11rp)
  [dis_z_est] -> Position Control1/12(DT_Z_O)
  [dis_x_est] -> Position Control1/13(DT_X_O)
  [dis_y_est] -> Position Control1/14(DT_Y_O)
  [x7rpp] -> Position Control1/5(x7rpp)
  [x9rpp] -> Position Control1/8(x9rpp)
  [x11rpp] -> Position Control1/11(x11rpp)
  Mux/1 -> Scope3/1

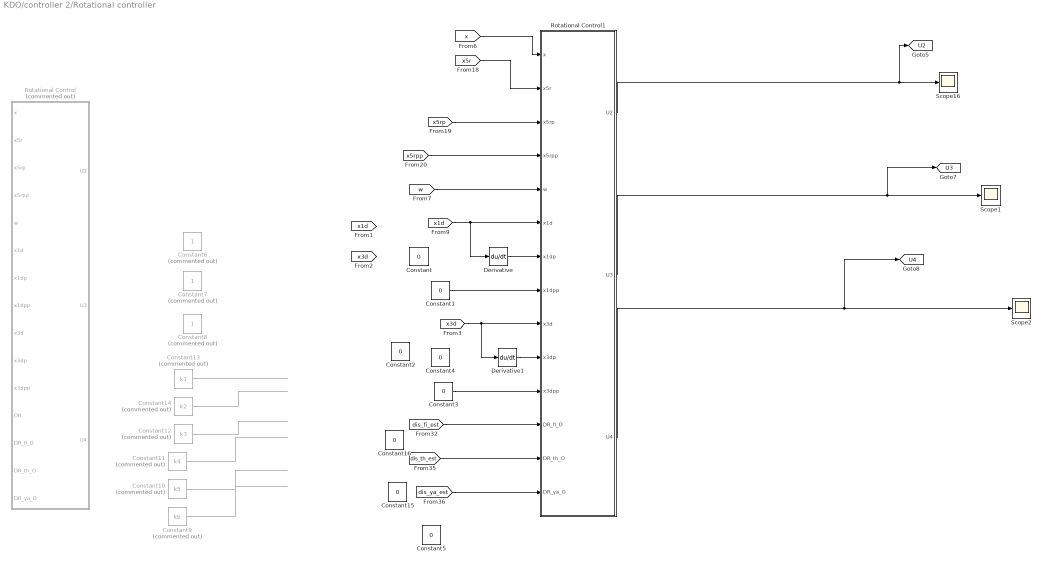
== system KDO/controller 2/Rotational controller  ==
  Constant{,1..5,15..16} (8 alike) : Constant  Value=0
  Constant10 : Constant  Commented=on  Value=k5
  Constant11 : Constant  Commented=on  Value=k4
  Constant12 : Constant  Commented=on  Value=k3
  Constant13 : Constant  Commented=on  Value=k1
  Constant14 : Constant  Commented=on  Value=k2
  Constant6 : Constant  Commented=on
  Constant7 : Constant  Commented=on
  Constant8 : Constant  Commented=on
  Constant9 : Constant  Commented=on  Value=k6
  Derivative : Derivative
  Derivative1 : Derivative
  Rotational Control : MATLAB Function  Commented=on  TreatAsAtomicUnit=on
  Rotational Control1 : MATLAB Function  TreatAsAtomicUnit=on
  Scope1 : Scope
  Scope16 : Scope
  Scope2 : Scope
  tag scope: U2=global, U3=global, U4=global
  wires:
  Rotational Control1/2(U3) -> Scope1/1, [U3]
  [x] -> Rotational Control1/1(x)
  [w] -> Rotational Control1/5(w)
  [x5rp] -> Rotational Control1/3(x5rp)
  Rotational Control1/3(U4) -> Scope2/1, [U4]
  [x5rpp] -> Rotational Control1/4(x5rpp)
  Rotational Control1/1(U2) -> Scope16/1, [U2]
  Constant1/1 -> Rotational Control1/8(x1dpp)
  Constant3/1 -> Rotational Control1/11(x3dpp)
  Constant13/1 -> ?
  Constant14/1 -> ?
  Constant12/1 -> ?
  Constant11/1 -> ?
  Constant10/1 -> ?
  Constant9/1 -> ?
  [x1d] -> Derivative/1, Rotational Control1/6(x1d)
  [x5r] -> Rotational Control1/2(x5r)
  [x3d] -> Derivative1/1, Rotational Control1/9(x3d)
  Derivative/1 -> Rotational Control1/7(x1dp)
  Derivative1/1 -> Rotational Control1/10(x3dp)
  [dis_fi_est] -> Rotational Control1/12(DR_fi_O)
  [dis_th_est] -> Rotational Control1/13(DR_th_O)
  [dis_ya_est] -> Rotational Control1/14(DR_ya_O)

== matlab function KDO/ Quadrotor plant #1 /MATLAB Function1 ==
  data: disR input; DR1 output; DR2 output; DR3 output
function [DR1,DR2,DR3]= fcn(disR)

Ix=2.098*10^-5;
Iy=2.12*10^-5;
Iz=3.269*10^-5;
l=39.73*10^-3;

DR1=disR(1)/Ix;
DR2=disR(2)/Iy;
DR3=disR(3)/Iz;

== matlab function KDO/ Quadrotor plant #1 /QR Plant  ==
  data: x_ input; w_ input; u_ input; dx output; DT input; DR input; uxa_ input; uya_ input
function dx = fcn(x_,w_,u_,DT,DR,uxa_,uya_)
%#eml 

%%  PARAMETERS   (According to paper #6)%%

U_=u_(1:4);

m=0.0296;
Ix=2.098*10^-5;
Iy=2.12*10^-5;
Iz=3.269*10^-5;
d=0.3;
g=9.81;
JR=(0.5*0.0025*23.1348*10^-3*23.1348*10^-3);
b=2.98*10^-5;
c=1.140*10^-7;
l=39.73*10^-3;

% m=1.83;
% Ix=21.6*10^-3;
% Iy=21.6*10^-3;
% Iz=43.2*10^-3;
% d=0.3;
% g=9.81;
% JR=3.357*10^-5;
% b=2.98*10^-5;
% c=1.140*10^-7;
% l=1;

a1=(Iy-Iz)/Ix;
a2=-JR/Ix;
a3=(Iz-Ix)/Iy;
a4=-JR/Iy;
a5=(Ix-Iy)/Iz;
b1=l/Ix;
b2=l/Iy;
b3=1/Iz;

%ux=cos(x(1))*sin(x(3))*cos(x(5))+sin(x(1))*sin(x(5));
%uy=cos(x(1))*sin(x(3))*sin(x(5))-sin(x(1))*cos(x(5));


dx1=x_(2);
dx2=x_(4)*x_(6)*a1+x_(4)*a2*w_+b1*U_(2)+DR(1);
dx3=x_(4);
dx4=x_(2)*x_(6)*a3+x_(2)*a4*w_+b2*U_(3)+DR(2);
dx5=x_(6);
dx6=x_(4)*x_(2)*a5+b3*U_(4)+DR(3);
dx7=x_(8);
dx8=-g+((1/m)*U_(1)*(cos(x_(1))*cos(x_(3))))+DT(1);
dx9=x_(10);
dx10=(uxa_/m)*U_(1)+DT(2);
dx11=x_(12);
dx12=(uya_/m)*U_(1)+DT(3);
     
dx=[dx1 dx2 dx3 dx4 dx5 dx6 dx7 dx8 dx9 dx10 dx11 dx12];
